simulink model "circuit2_simulink"  (R2014a)
settings: Solver=ode45  StartTime=0.0  StopTime=60.0  FixedStep=0.0001  RelTol=1e-3
undefined symbols (not defined in the file): C, L, R
settings Model: Creator=emilio  LastModifiedBy=emilio

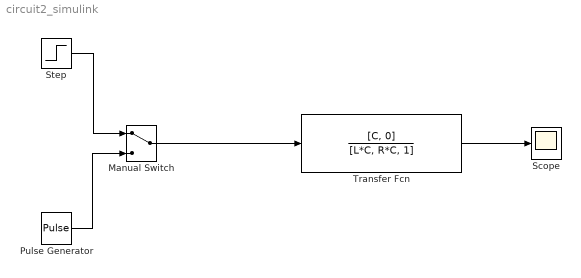
== system circuit2_simulink ==
  Manual Switch : ManualSwitch  SampleTime=0.001
  Pulse Generator : DiscretePulseGenerator  PulseType=Time based  Period=30  PulseWidth=50  PhaseDelay=15
  Scope : Scope
      settings: TimeRange=10
  Step : Step  SampleTime=.01
  Transfer Fcn : TransferFcn  Numerator=[C, 0]  Denominator=[L*C, R*C, 1]
  wires:
  Step/1 -> Manual Switch/1
  Manual Switch/1 -> Transfer Fcn/1
  Pulse Generator/1 -> Manual Switch/2
  Transfer Fcn/1 -> Scope/1
